simulink model "lightsoccer"  (R2016b)
settings: Solver=VariableStepDiscrete  StartTime=0.0  StopTime=1.8  FixedStep=.15  RelTol=1e-3
values from neighbouring files (symbols this model uses):
  K_lqr2 = lqr(sysdrect2,Q2,R1,0)    [LQR.m]
  sysdopt = sysdeul    [setpoints.m]
  Ts = double(subs(Ts))    [dstatespace.m]    (also in dynamickeep.m = 0.15)
  x0 = [0;0;0;0;0;0]    [Copy_of_MPC.m]    (also in LQR.m; MPC.m; optimkeeper.m = [1,1,1]; setpoints.m)
settings Model: Creator=r0610649  LastModifiedBy=r0610649

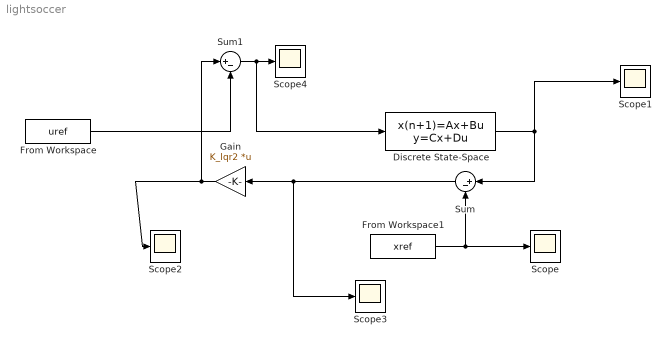
== system lightsoccer ==
  Discrete State-Space : DiscreteStateSpace  A=sysdopt.A  B=sysdopt.B  C=sysdopt.C  D=sysdopt.D  X0=x0  SampleTime=Ts
  From Workspace : FromWorkspace  VariableName=uref  SampleTime=.15  Interpolate=off  OutputAfterFinalValue=Holding final value
  From Workspace1 : FromWorkspace  VariableName=xref  SampleTime=.15  Interpolate=off  OutputAfterFinalValue=Holding final value
  Gain : Gain  Gain=K_lqr2  Multiplication=Matrix(K*u)
  Scope{,1..4} (5 alike) : Scope
  Sum : Sum  Inputs=|+-
  Sum1 : Sum  Inputs=|+-
  wires:
  Discrete State-Space/1 -> Sum/1, Scope1/1
  From Workspace1/1 -> Sum/2, Scope/1
  Gain/1 -> Scope2/1, Sum1/1
  From Workspace/1 -> Sum1/2
  Sum/1 -> Scope3/1, Gain/1
  Sum1/1 -> Discrete State-Space/1, Scope4/1
